simulink model "quadrocopter_controller"  (Simulink 7.4)
settings: Solver=ode45  StartTime=0.0  StopTime=50  RelTol=1e-3
values from neighbouring files (symbols this model uses):
  g = 9.81    [quadrocopter_param.m]
  I_x = elec.I_x+bat.I_x+2*boom.I_1x+2*boom.I_1y+2*mot.I_1x+2*mot.I_1y+                             2*rot.I_1x+2*rot.I_1y    [quadrocopter_param.m]
  I_y = elec.I_y+bat.I_y+2*boom.I_1x+2*boom.I_1y+2*mot.I_1x+2*mot.I_1y+                             2*rot.I_1x+2*rot.I_1y    [quadrocopter_param.m]
  I_z = elec.I_z+bat.I_z+4*boom.I_1z+4*mot.I_1x+4*rot.I_1x    [quadrocopter_param.m]
  m = elec.m+bat.m+boom.m+mot.m+rot.m    [quadrocopter_param.m]
undefined symbols (not defined in the file or in its folder): boom
libraries: simulink x12
settings Model: Creator=Sreekanth  LastModifiedBy=Joachim
settings DebuggingCC: SolverPrmCheckMsg=none

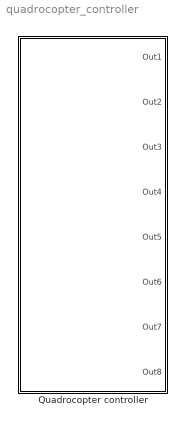
== system quadrocopter_controller ==
  Quadrocopter controller : Subsystem

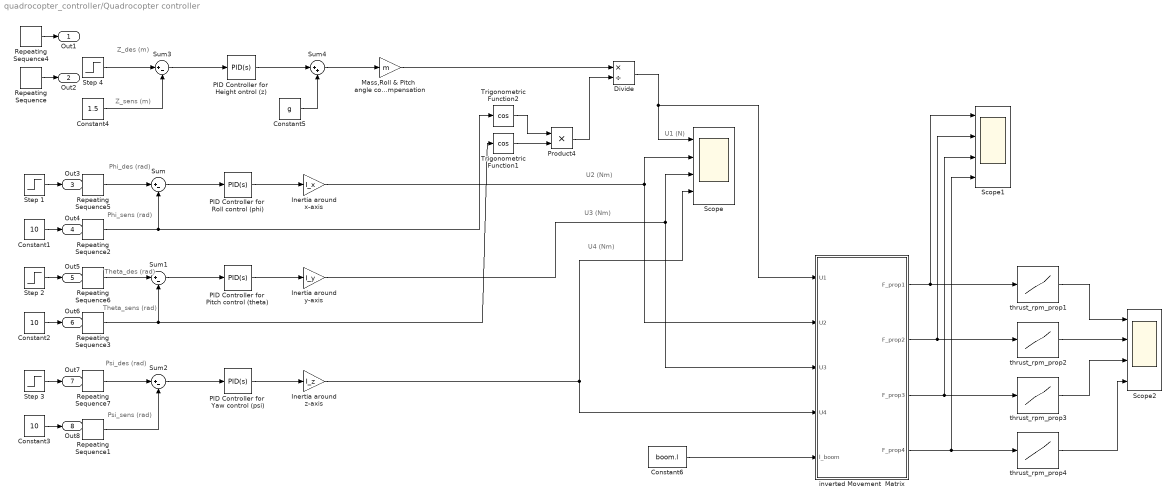
== system quadrocopter_controller/Quadrocopter controller ==
  note: Phi_des (rad)
  note: Phi_sens (rad)
  note: Theta_des (rad)
  note: Theta_sens (rad)
  note: Psi_des (rad)
  note: Psi_sens (rad)
  note: Z_des (m)
  note: Z_sens (m)
  note: U2 (Nm)
  note: U3 (Nm)
  note: U4 (Nm)
  note: U1 (N)
  Constant1 : Constant  Value=10  OutDataType=fixdt(1, 16)  OutScaling=2^0
  Constant2 : Constant  Value=10  OutDataType=fixdt(1, 16)  OutScaling=2^0
  Constant3 : Constant  Value=10  OutDataType=fixdt(1, 16)  OutScaling=2^0
  Constant4 : Constant  Value=1.5  OutDataType=fixdt(1, 16)  OutScaling=2^0
  Constant5 : Constant  Value=g  OutDataType=fixdt(1, 16)  OutScaling=2^0
  Constant6 : Constant  Value=boom.l  OutDataType=fixdt(1, 16)  OutScaling=2^0
  Divide : Product  Inputs=*/  OutDataType=fixdt(1, 16)  OutScaling=2^-10
  Inertia around x-axis : Gain  Gain=I_x  ParameterDataType=fixdt(1, 16)  ParameterScaling=2^0  OutDataType=fixdt(1, 16)  OutScaling=2^0
  Inertia around y-axis : Gain  Gain=I_y  ParameterDataType=fixdt(1, 16)  ParameterScaling=2^0  OutDataType=fixdt(1, 16)  OutScaling=2^0
  Inertia around z-axis : Gain  Gain=I_z  ParameterDataType=fixdt(1, 16)  ParameterScaling=2^0  OutDataType=fixdt(1, 16)  OutScaling=2^0
  Mass,Roll & Pitch  angle compensation : Gain  Gain=m  ParameterDataType=fixdt(1, 16)  ParameterScaling=2^0  OutDataType=fixdt(1, 16)  OutScaling=2^0
  PID Controller for  Height ontrol (z) : simulink/Continuous/PID Controller  DialogController=pidpack.PIDConfig.pidDDGCreate  DialogControllerArgs=DataTag0  SystemSampleTime=-1  Controller=PID  TimeDomain=Continuous-time  SampleTime=1  IntegratorMethod=Forward Euler  FilterMethod=Forward Euler  Form=Parallel  P=1  I=1  D=0  N=100  InitialConditionSource=internal  InitialConditionForIntegrator=0  InitialConditionForFilter=0  ExternalReset=none  LimitOutput=on  UpperSaturationLimit=20  LowerSaturationLimit=0  LinearizeAsGain=off  AntiWindupMode=clamping  Kb=1  TrackingMode=off  Kt=1  PParamMin=[]  PParamMax=[]  IParamMin=[]  IParamMax=[]  DParamMin=[]  DParamMax=[]  NParamMin=[]  NParamMax=[]  KbParamMin=[]  KbParamMax=[]  KtParamMin=[]  KtParamMax=[]  POutMin=[]  POutMax=[]  IOutMin=[]  IOutMax=[]  DOutMin=[]  DOutMax=[]  NOutMin=[]  NOutMax=[]  KbOutMin=[]  KbOutMax=[]  KtOutMin=[]  KtOutMax=[]  IntegratorOutMin=[]  IntegratorOutMax=[]  FilterOutMin=[]  FilterOutMax=[]  SumOutMin=[]  SumOutMax=[]  SumI1OutMin=[]  SumI1OutMax=[]  SumI2OutMin=[]  SumI2OutMax=[]  SumI3OutMin=[]  SumI3OutMax=[]  SumDOutMin=[]  SumDOutMax=[]  SaturationOutMin=[]  SaturationOutMax=[]  IntegratorContinuousStateAttributes=''  IntegratorStateMustResolveToSignalObject=off  IntegratorRTWStateStorageClass=Auto  FilterContinuousStateAttributes=''  FilterStateMustResolveToSignalObject=off  FilterRTWStateStorageClass=Auto
  PID Controller for  Pitch control (theta) : simulink/Continuous/PID Controller  DialogController=pidpack.PIDConfig.pidDDGCreate  DialogControllerArgs=DataTag1  SystemSampleTime=-1  Controller=PID  TimeDomain=Continuous-time  SampleTime=1  IntegratorMethod=Forward Euler  FilterMethod=Forward Euler  Form=Parallel  P=1000  I=10  D=0  N=100  InitialConditionSource=internal  InitialConditionForIntegrator=0  InitialConditionForFilter=0  ExternalReset=none  LimitOutput=on  UpperSaturationLimit=20  LowerSaturationLimit=-20  LinearizeAsGain=off  AntiWindupMode=clamping  Kb=1  TrackingMode=off  Kt=1  PParamMin=[]  PParamMax=[]  IParamMin=[]  IParamMax=[]  DParamMin=[]  DParamMax=[]  NParamMin=[]  NParamMax=[]  KbParamMin=[]  KbParamMax=[]  KtParamMin=[]  KtParamMax=[]  POutMin=[]  POutMax=[]  IOutMin=[]  IOutMax=[]  DOutMin=[]  DOutMax=[]  NOutMin=[]  NOutMax=[]  KbOutMin=[]  KbOutMax=[]  KtOutMin=[]  KtOutMax=[]  IntegratorOutMin=[]  IntegratorOutMax=[]  FilterOutMin=[]  FilterOutMax=[]  SumOutMin=[]  SumOutMax=[]  SumI1OutMin=[]  SumI1OutMax=[]  SumI2OutMin=[]  SumI2OutMax=[]  SumI3OutMin=[]  SumI3OutMax=[]  SumDOutMin=[]  SumDOutMax=[]  SaturationOutMin=[]  SaturationOutMax=[]  IntegratorContinuousStateAttributes=''  IntegratorStateMustResolveToSignalObject=off  IntegratorRTWStateStorageClass=Auto  FilterContinuousStateAttributes=''  FilterStateMustResolveToSignalObject=off  FilterRTWStateStorageClass=Auto
  PID Controller for  Roll control (phi) : simulink/Continuous/PID Controller  DialogController=pidpack.PIDConfig.pidDDGCreate  DialogControllerArgs=DataTag2  SystemSampleTime=-1  Controller=PID  TimeDomain=Continuous-time  SampleTime=1  IntegratorMethod=Forward Euler  FilterMethod=Forward Euler  Form=Parallel  P=1000  I=10  D=0  N=100  InitialConditionSource=internal  InitialConditionForIntegrator=0  InitialConditionForFilter=0  ExternalReset=none  LimitOutput=on  UpperSaturationLimit=20  LowerSaturationLimit=-20  LinearizeAsGain=off  AntiWindupMode=clamping  Kb=1  TrackingMode=off  Kt=1  PParamMin=[]  PParamMax=[]  IParamMin=[]  IParamMax=[]  DParamMin=[]  DParamMax=[]  NParamMin=[]  NParamMax=[]  KbParamMin=[]  KbParamMax=[]  KtParamMin=[]  KtParamMax=[]  POutMin=[]  POutMax=[]  IOutMin=[]  IOutMax=[]  DOutMin=[]  DOutMax=[]  NOutMin=[]  NOutMax=[]  KbOutMin=[]  KbOutMax=[]  KtOutMin=[]  KtOutMax=[]  IntegratorOutMin=[]  IntegratorOutMax=[]  FilterOutMin=[]  FilterOutMax=[]  SumOutMin=[]  SumOutMax=[]  SumI1OutMin=[]  SumI1OutMax=[]  SumI2OutMin=[]  SumI2OutMax=[]  SumI3OutMin=[]  SumI3OutMax=[]  SumDOutMin=[]  SumDOutMax=[]  SaturationOutMin=[]  SaturationOutMax=[]  IntegratorContinuousStateAttributes=''  IntegratorStateMustResolveToSignalObject=off  IntegratorRTWStateStorageClass=Auto  FilterContinuousStateAttributes=''  FilterStateMustResolveToSignalObject=off  FilterRTWStateStorageClass=Auto
  PID Controller for  Yaw control (psi) : simulink/Continuous/PID Controller  DialogController=pidpack.PIDConfig.pidDDGCreate  DialogControllerArgs=DataTag3  SystemSampleTime=-1  Controller=PID  TimeDomain=Continuous-time  SampleTime=1  IntegratorMethod=Forward Euler  FilterMethod=Forward Euler  Form=Parallel  P=1000  I=10  D=0  N=100  InitialConditionSource=internal  InitialConditionForIntegrator=0  InitialConditionForFilter=0  ExternalReset=none  LimitOutput=on  UpperSaturationLimit=180  LowerSaturationLimit=-180  LinearizeAsGain=off  AntiWindupMode=clamping  Kb=1  TrackingMode=off  Kt=1  PParamMin=[]  PParamMax=[]  IParamMin=[]  IParamMax=[]  DParamMin=[]  DParamMax=[]  NParamMin=[]  NParamMax=[]  KbParamMin=[]  KbParamMax=[]  KtParamMin=[]  KtParamMax=[]  POutMin=[]  POutMax=[]  IOutMin=[]  IOutMax=[]  DOutMin=[]  DOutMax=[]  NOutMin=[]  NOutMax=[]  KbOutMin=[]  KbOutMax=[]  KtOutMin=[]  KtOutMax=[]  IntegratorOutMin=[]  IntegratorOutMax=[]  FilterOutMin=[]  FilterOutMax=[]  SumOutMin=[]  SumOutMax=[]  SumI1OutMin=[]  SumI1OutMax=[]  SumI2OutMin=[]  SumI2OutMax=[]  SumI3OutMin=[]  SumI3OutMax=[]  SumDOutMin=[]  SumDOutMax=[]  SaturationOutMin=[]  SaturationOutMax=[]  IntegratorContinuousStateAttributes=''  IntegratorStateMustResolveToSignalObject=off  IntegratorRTWStateStorageClass=Auto  FilterContinuousStateAttributes=''  FilterStateMustResolveToSignalObject=off  FilterRTWStateStorageClass=Auto
  Product4 : Product  OutDataType=fixdt(1, 16)  OutScaling=2^0  RndMeth=Zero
  Repeating Sequence : simulink/Sources/Repeating Sequence  SystemSampleTime=-1  rep_seq_t=[0 1 2 3 4 5 6 7 8 9 10]  rep_seq_y=[17 17 17 17 18 18 18 19 19 19 19]
  Repeating Sequence1 : simulink/Sources/Repeating Sequence  SystemSampleTime=-1  rep_seq_t=[0 1 2 3 4 5 6 7 8 9 10]  rep_seq_y=[1 1 1 1 1 1 1 1 1 1 1]
  Repeating Sequence2 : simulink/Sources/Repeating Sequence  SystemSampleTime=-1  rep_seq_t=[0 1 2 3 4 5 6 7 8 9 10]  rep_seq_y=[1 1 1 1 1 1 1 1 1 1 1]
  Repeating Sequence3 : simulink/Sources/Repeating Sequence  SystemSampleTime=-1  rep_seq_t=[0 1 2 3 4 5 6 7 8 9 10]  rep_seq_y=[1 1 1 1 1 1 1 1 1 1 1]
  Repeating Sequence4 : simulink/Sources/Repeating Sequence  SystemSampleTime=-1  rep_seq_t=[0 1 2 3 4 5 6 7 8 9 10]  rep_seq_y=[34 34 34 34 36 36 36 38 38 38 38]
  Repeating Sequence5 : simulink/Sources/Repeating Sequence  SystemSampleTime=-1  rep_seq_t=[0 1 2 3 4 5 6 7 8 9 10]  rep_seq_y=[1 0 1 0 1 0 1 0 1 0 1]
  Repeating Sequence6 : simulink/Sources/Repeating Sequence  SystemSampleTime=-1  rep_seq_t=[0 1 2 3 4 5 6 7 8 9 10]  rep_seq_y=[1 0 1 0 1 0 1 0 1 0 1]
  Repeating Sequence7 : simulink/Sources/Repeating Sequence  SystemSampleTime=-1  rep_seq_t=[0 1 2 3 4 5 6 7 8 9 10]  rep_seq_y=[1 0 1 0 1 0 1 0 1 0 1]
  Scope : Scope  NumInputPorts=4
      settings: TimeRange=10  YMin=16.5147~0.359533~0.366931~0.234953  YMax=16.5153~0.397379~0.366932~0.259685
  Scope1 : Scope  NumInputPorts=4
      settings: TimeRange=10  YMin=-5~-5~-5~-5  YMax=5~5~5~5
  Scope2 : Scope  NumInputPorts=4
      settings: TimeRange=10  YMin=0~0~0~0  YMax=10000~10000~10000~10000  SaveName=ScopeData2
  Step 1 : Step  After=20  SampleTime=0
  Step 2 : Step  After=20  SampleTime=0
  Step 3 : Step  After=20  SampleTime=0
  Step 4 : Step  After=2  SampleTime=0
  Sum{,1..3} (4 alike) : Sum  Inputs=|+-  OutDataType=fixdt(1, 16)  OutScaling=2^0
  Sum4 : Sum  Inputs=|++  OutDataType=fixdt(1, 16)  OutScaling=2^0
  Trigonometric Function1 : Trigonometry  Operator=cos
  Trigonometric Function2 : Trigonometry  Operator=cos
  inverted Movement  Matrix : Stateflow chart
  thrust_rpm_prop{1..4} (4 alike) : Lookup  InputValues=[0.58 1 1.33 2 2.54 3.33 4.08 4.54]  Table=[1988 2544 2940 3566 4033 4500 5033 5233]  OutDataType=fixdt(1, 16)  OutScaling=2^0
  Out1 : Outport
  Out2 : Outport  Port=2
  Out3 : Outport  Port=3
  Out4 : Outport  Port=4
  Out5 : Outport  Port=5
  Out6 : Outport  Port=6
  Out7 : Outport  Port=7
  Out8 : Outport  Port=8
  wires:
  Sum/1 -> PID Controller for  Roll control (phi)/1
  Sum1/1 -> PID Controller for  Pitch control (theta)/1
  Sum2/1 -> PID Controller for  Yaw control (psi)/1
  PID Controller for  Roll control (phi)/1 -> Inertia around x-axis/1
  PID Controller for  Pitch control (theta)/1 -> Inertia around y-axis/1
  PID Controller for  Yaw control (psi)/1 -> Inertia around z-axis/1
  Sum3/1 -> PID Controller for  Height ontrol (z)/1
  Sum4/1 -> Mass,Roll & Pitch  angle compensation/1
  Constant5/1 -> Sum4/2
  Trigonometric Function2/1 -> Product4/1
  Trigonometric Function1/1 -> Product4/2
  Product4/1 -> Divide/2
  Divide/1 -> Scope/1, inverted Movement  Matrix/1(U1)
  Inertia around y-axis/1 -> Scope/3, inverted Movement  Matrix/3(U3)
  Inertia around z-axis/1 -> Scope/4, inverted Movement  Matrix/4(U4)
  PID Controller for  Height ontrol (z)/1 -> Sum4/1
  Mass,Roll & Pitch  angle compensation/1 -> Divide/1
  Constant6/1 -> inverted Movement  Matrix/5(l_boom)
  thrust_rpm_prop1/1 -> Scope2/1
  thrust_rpm_prop3/1 -> Scope2/3
  thrust_rpm_prop4/1 -> Scope2/4
  Inertia around x-axis/1 -> Scope/2, inverted Movement  Matrix/2(U2)
  inverted Movement  Matrix/1(F_prop1) -> Scope1/1, thrust_rpm_prop1/1
  inverted Movement  Matrix/2(F_prop2) -> Scope1/2, thrust_rpm_prop2/1
  inverted Movement  Matrix/3(F_prop3) -> Scope1/3, thrust_rpm_prop3/1
  inverted Movement  Matrix/4(F_prop4) -> Scope1/4, thrust_rpm_prop4/1
  thrust_rpm_prop2/1 -> Scope2/2
  Repeating Sequence2/1 -> Trigonometric Function2/1, Sum/2
  Repeating Sequence1/1 -> Sum2/2
  Repeating Sequence3/1 -> Trigonometric Function1/1, Sum1/2
  Repeating Sequence5/1 -> Sum/1
  Repeating Sequence6/1 -> Sum1/1
  Repeating Sequence7/1 -> Sum2/1
  Step 4/1 -> Sum3/1
  Constant4/1 -> Sum3/2
  Repeating Sequence4/1 -> Out1/1
  Repeating Sequence/1 -> Out2/1
  Step 1/1 -> Out3/1
  Constant1/1 -> Out4/1
  Step 2/1 -> Out5/1
  Constant2/1 -> Out6/1
  Step 3/1 -> Out7/1
  Constant3/1 -> Out8/1

== matlab function Quadrocopter controller/inverted Movement Matrix ==
  data: U1 input double; F_prop1 output double; F_prop2 output double; F_prop3 output double; F_prop4 output double; U2 input double; U3 input double; U4 input double; l_boom input double
function [F_prop1,F_prop2,F_prop3,F_prop4] = fcn(U1,U2,U3,U4,l_boom)
%#eml

% Force needed at the front propeller in [N]
F_prop1 = (U1/4)-(U3/(2*l_boom))+(U4/(4*l_boom));

% Force needed at the left propeller in [N]
F_prop2 = (U1/4)+(U2/(2*l_boom))-(U4/(4*l_boom));

% Force needed at the back propeller in [N]
F_prop3 = (U1/4)+(U3/(2*l_boom))+(U4/(4*l_boom));

% Force needed at the right propeller in [N]
F_prop4 = (U1/4)-(U2/(2*l_boom))-(U4/(4*l_boom));
